simulink model "Euler_Quaternion"  (Simulink 7.9)
settings: Solver=ode45  StartTime=0.0  StopTime=10.0  RelTol=1e-3
undefined symbols (not defined in the file or in its folder): Newton, nfs, Raphson
libraries: aerolibanim x1, aerolibutil x1
settings Model: Creator=AHKh PC  LastModifiedBy=AHKh PC

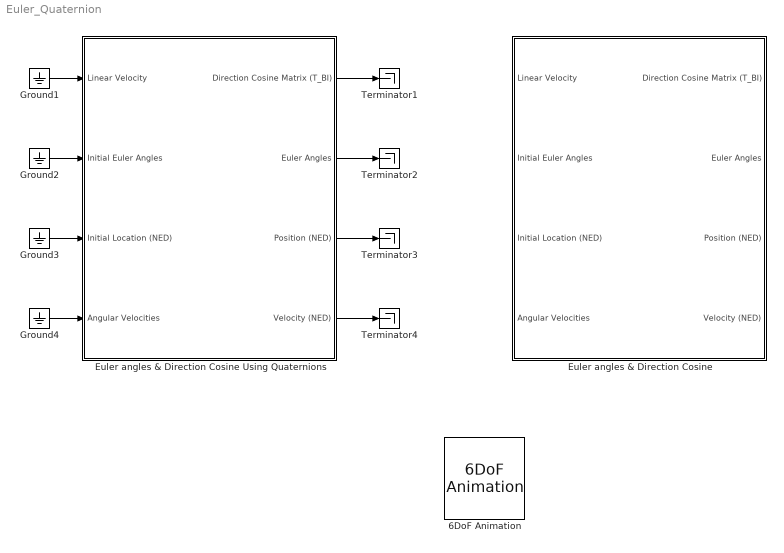
== system Euler_Quaternion ==
  6DoF Animation : aerolibanim/6DoF Animation  u1=[0 4000 -2000 2000 -5000 -3000]  u2=0.1  u3=1000.0  u4=[4000 0 -5000]  u5=Fly alongside  u6=[0 500 0]  u7=100  u8=on
  Euler angles & Direction Cosine : Subsystem
  Euler angles & Direction Cosine Using Quaternions : Subsystem
  Ground{1..4} (4 alike) : Ground
  Terminator{1..4} (4 alike) : Terminator
  wires:
  Euler angles & Direction Cosine Using Quaternions/1(Direction Cosine Matrix (T_BI)) -> Terminator1/1
  Euler angles & Direction Cosine Using Quaternions/2(Euler Angles) -> Terminator2/1
  Euler angles & Direction Cosine Using Quaternions/3(Position (NED)) -> Terminator3/1
  Euler angles & Direction Cosine Using Quaternions/4(Velocity (NED)) -> Terminator4/1
  Ground1/1 -> Euler angles & Direction Cosine Using Quaternions/1(Linear Velocity)
  Ground2/1 -> Euler angles & Direction Cosine Using Quaternions/2(Initial Euler Angles)
  Ground3/1 -> Euler angles & Direction Cosine Using Quaternions/3(Initial Location (NED))
  Ground4/1 -> Euler angles & Direction Cosine Using Quaternions/4(Angular Velocities)

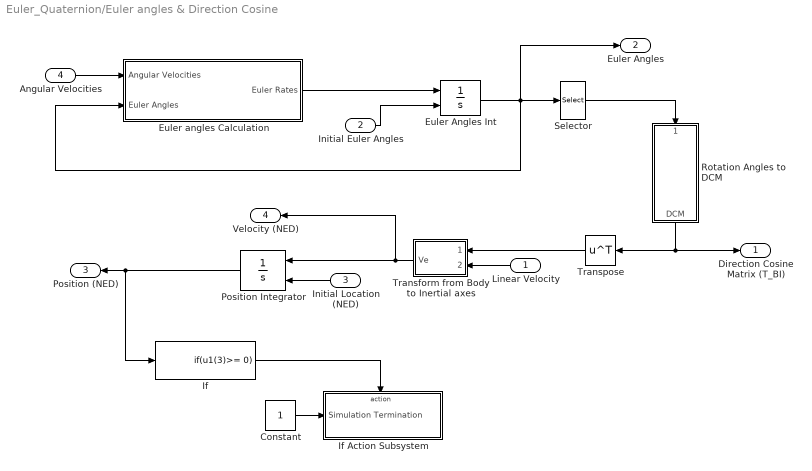
== system Euler_Quaternion/Euler angles & Direction Cosine ==
  Linear Velocity : Inport  PortDimensions=[3,1]
  Initial Euler Angles : Inport  Port=2
  Initial Location (NED) : Inport  Port=3  PortDimensions=[3,1]
  Angular Velocities : Inport  Port=4
  Constant : Constant
  Euler Angles Int : Integrator  InitialConditionSource=external  InitialCondition=nfs.attitude0
  Euler angles Calculation : Subsystem
  If : If  IfExpression=u1(3)>= 0  ShowElse=off
  If Action Subsystem : Subsystem  TreatAsAtomicUnit=on
  Position Integrator : Integrator  InitialConditionSource=external  InitialCondition=[0,0,nfs.attitude0]
  Rotation Angles to DCM : Subsystem
  Selector : Selector  InputPortWidth=3  IndexOptions=Index vector (dialog)  Indices=[3 2 1]  OutputSizes=1
  Transform from Body to Inertial axes : Subsystem
      mask Display: disp('T_IB')
  Transpose : Math  Operator=transpose  SaturateOnIntegerOverflow=on
  Direction Cosine Matrix (T_BI) : Outport  PortDimensions=[3,3]
  Euler Angles : Outport  Port=2
  Position (NED) : Outport  Port=3  PortDimensions=[3,1]
  Velocity (NED) : Outport  Port=4  PortDimensions=[3,1]
  wires:
  Initial Euler Angles/1 -> Euler Angles Int/2
  Rotation Angles to DCM/1(DCM) -> Transpose/1, Direction Cosine Matrix (T_BI)/1
  Angular Velocities/1 -> Euler angles Calculation/1(Angular Velocities)
  Selector/1 -> Rotation Angles to DCM/1("[R1,R2,R3]")
  Transpose/1 -> Transform from Body to Inertial axes/1(Transformation Matrix)
  Linear Velocity/1 -> Transform from Body to Inertial axes/2(Position Vector)
  Initial Location (NED)/1 -> Position Integrator/2
  Euler Angles Int/1 -> Euler Angles/1, Selector/1, Euler angles Calculation/2(Euler Angles)
  Transform from Body to Inertial axes/1(Ve) -> Velocity (NED)/1, Position Integrator/1
  Position Integrator/1 -> Position (NED)/1, If/1
  Euler angles Calculation/1(Euler Rates) -> Euler Angles Int/1
  If/1 -> If Action Subsystem/Action
  Constant/1 -> If Action Subsystem/1(Simulation Termination)

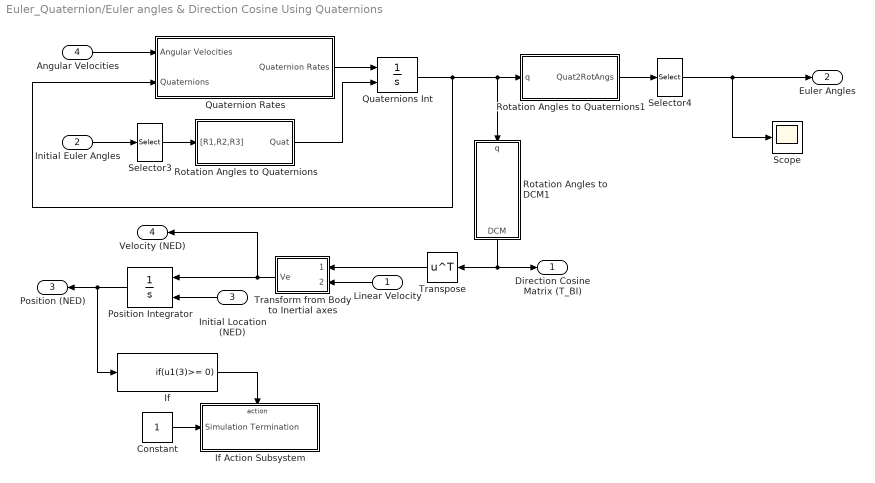
== system Euler_Quaternion/Euler angles & Direction Cosine Using Quaternions ==
  Linear Velocity : Inport  PortDimensions=[3,1]
  Initial Euler Angles : Inport  Port=2  PortDimensions=[3,1]
  Initial Location (NED) : Inport  Port=3  PortDimensions=[3,1]
  Angular Velocities : Inport  Port=4  PortDimensions=[3,1]
  Constant : Constant
  If : If  IfExpression=u1(3)>= 0  ShowElse=off
  If Action Subsystem : Subsystem  TreatAsAtomicUnit=on
  Position Integrator : Integrator  InitialConditionSource=external  InitialCondition=[0,0,nfs.attitude0]
  Quaternion Rates : Subsystem
  Quaternions Int : Integrator  InitialConditionSource=external  InitialCondition=nfs.attitude0  ContinuousStateAttributes='Quaternions'
  Rotation Angles to DCM1 : Subsystem
  Rotation Angles to Quaternions : Subsystem
  Rotation Angles to Quaternions1 : Subsystem
  Scope : Scope
      settings: SaveName=ScopeData23
  Selector3 : Selector  InputPortWidth=3  IndexOptions=Index vector (dialog)  Indices=[3 2 1]  OutputSizes=1
  Selector4 : Selector  InputPortWidth=3  IndexOptions=Index vector (dialog)  Indices=[3 2 1]  OutputSizes=1
  Transform from Body to Inertial axes : Subsystem
      mask Display: disp('T_IB')
  Transpose : Math  Operator=transpose  SaturateOnIntegerOverflow=on
  Direction Cosine Matrix (T_BI) : Outport  PortDimensions=[3,3]
  Euler Angles : Outport  Port=2  PortDimensions=[3,1]
  Position (NED) : Outport  Port=3  PortDimensions=[3,1]
  Velocity (NED) : Outport  Port=4  PortDimensions=[3,1]
  wires:
  Position Integrator/1 -> Position (NED)/1, If/1
  Transform from Body to Inertial axes/1(Ve) -> Position Integrator/1, Velocity (NED)/1
  Initial Location (NED)/1 -> Position Integrator/2
  Linear Velocity/1 -> Transform from Body to Inertial axes/2(Position Vector)
  Transpose/1 -> Transform from Body to Inertial axes/1(Transformation Matrix)
  Quaternion Rates/1(Quaternion Rates) -> Quaternions Int/1
  Angular Velocities/1 -> Quaternion Rates/1(Angular Velocities)
  Initial Euler Angles/1 -> Selector3/1
  Selector3/1 -> Rotation Angles to Quaternions/1("[R1,R2,R3]")
  Rotation Angles to Quaternions/1(Quat) -> Quaternions Int/2
  Quaternions Int/1 -> Quaternion Rates/2(Quaternions), Rotation Angles to Quaternions1/1(q), Rotation Angles to DCM1/1(q)
  Rotation Angles to Quaternions1/1(Quat2RotAngs) -> Selector4/1
  Selector4/1 -> Euler Angles/1, Scope/1
  Rotation Angles to DCM1/1(DCM) -> Direction Cosine Matrix (T_BI)/1, Transpose/1
  Constant/1 -> If Action Subsystem/1(Simulation Termination)
  If/1 -> If Action Subsystem/Action

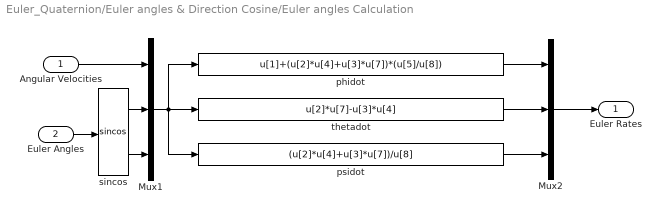
== system Euler_Quaternion/Euler angles & Direction Cosine/Euler angles Calculation ==
  Angular Velocities : Inport  PortDimensions=[3,1]
  Euler Angles : Inport  Port=2
  Mux1 : Mux  Inputs=[3 3 3]
  Mux2 : Mux  Inputs=3
  phidot : Fcn  Expr=u[1]+(u[2]*u[4]+u[3]*u[7])*(u[5]/u[8])
  psidot : Fcn  Expr=(u[2]*u[4]+u[3]*u[7])/u[8]
  sincos : Trigonometry  Operator=sincos
  thetadot : Fcn  Expr=u[2]*u[7]-u[3]*u[4]
  Euler Rates : Outport  PortDimensions=[3,1]  InitialOutput=0
  wires:
  sincos/2 -> Mux1/3
  sincos/1 -> Mux1/2
  Mux2/1 -> Euler Rates/1
  phidot/1 -> Mux2/1
  thetadot/1 -> Mux2/2
  psidot/1 -> Mux2/3
  Euler Angles/1 -> sincos/1
  Angular Velocities/1 -> Mux1/1
  Mux1/1 -> psidot/1, phidot/1, thetadot/1

== system Euler_Quaternion/Euler angles & Direction Cosine/If Action Subsystem ==
  Simulation Termination : Inport
  Action Port : ActionPort
  Stop Simulation : Stop
  wires:
  Simulation Termination/1 -> Stop Simulation/1

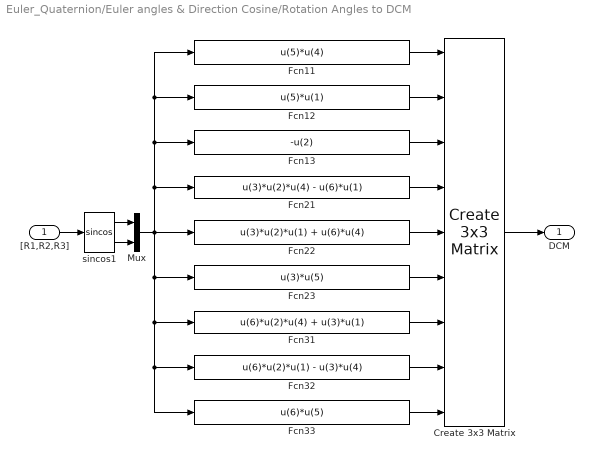
== system Euler_Quaternion/Euler angles & Direction Cosine/Rotation Angles to DCM ==
  "[R1,R2,R3]" : Inport  PortDimensions=3
  Create 3x3 Matrix : aerolibutil/Create 3x3 Matrix
  Fcn11 : Fcn  Expr=u(5)*u(4)
  Fcn12 : Fcn  Expr=u(5)*u(1)
  Fcn13 : Fcn  Expr=-u(2)
  Fcn21 : Fcn  Expr=u(3)*u(2)*u(4) - u(6)*u(1)
  Fcn22 : Fcn  Expr=u(3)*u(2)*u(1) + u(6)*u(4)
  Fcn23 : Fcn  Expr=u(3)*u(5)
  Fcn31 : Fcn  Expr=u(6)*u(2)*u(4) + u(3)*u(1)
  Fcn32 : Fcn  Expr=u(6)*u(2)*u(1) - u(3)*u(4)
  Fcn33 : Fcn  Expr=u(6)*u(5)
  Mux : Mux  Inputs=2
  sincos1 : Trigonometry  Operator=sincos
  DCM : Outport  PortDimensions=[3,3]
  wires:
  "[R1,R2,R3]"/1 -> sincos1/1
  Create 3x3 Matrix/1 -> DCM/1
  sincos1/1 -> Mux/1
  sincos1/2 -> Mux/2
  Mux/1 -> Fcn32/1, Fcn33/1, Fcn31/1, Fcn23/1, Fcn22/1, Fcn11/1, Fcn12/1, Fcn13/1, Fcn21/1
  Fcn11/1 -> Create 3x3 Matrix/1
  Fcn12/1 -> Create 3x3 Matrix/2
  Fcn13/1 -> Create 3x3 Matrix/3
  Fcn21/1 -> Create 3x3 Matrix/4
  Fcn31/1 -> Create 3x3 Matrix/7
  Fcn22/1 -> Create 3x3 Matrix/5
  Fcn23/1 -> Create 3x3 Matrix/6
  Fcn32/1 -> Create 3x3 Matrix/8
  Fcn33/1 -> Create 3x3 Matrix/9

== system Euler_Quaternion/Euler angles & Direction Cosine/Transform from Body to Inertial axes ==
  Transformation Matrix : Inport
  Position Vector : Inport  Port=2
  Product : Product  Multiplication=Matrix(*)  SaturateOnIntegerOverflow=on  InputSameDT=on  OutDataTypeStr=Inherit: Same as first input
  Reshape1 : Reshape  OutputDimensionality=Column vector (2-D)
  Reshape2 : Reshape
  Ve : Outport
  wires:
  Reshape2/1 -> Ve/1
  Reshape1/1 -> Product/2
  Position Vector/1 -> Reshape1/1
  Transformation Matrix/1 -> Product/1
  Product/1 -> Reshape2/1

== system Euler_Quaternion/Euler angles & Direction Cosine Using Quaternions/If Action Subsystem ==
  Simulation Termination : Inport
  Action Port : ActionPort  ActionType=then
  Stop Simulation : Stop
  wires:
  Simulation Termination/1 -> Stop Simulation/1

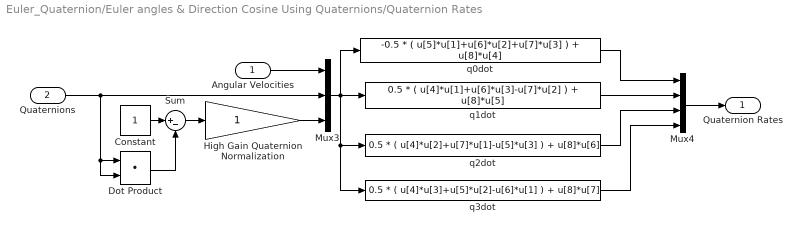
== system Euler_Quaternion/Euler angles & Direction Cosine Using Quaternions/Quaternion Rates ==
  Angular Velocities : Inport  PortDimensions=[3,1]
  Quaternions : Inport  Port=2  PortDimensions=4
  Constant : Constant
  Dot Product : DotProduct  OutDataTypeStr=Inherit: Inherit via internal rule
  High Gain Quaternion Normalization : Gain  SaturateOnIntegerOverflow=on  OutDataTypeStr=Inherit: Same as input  ParamDataTypeStr=Inherit: Same as input
  Mux3 : Mux  Inputs=[3 4 1]
  Mux4 : Mux
  Sum : Sum  Inputs=|+-  SaturateOnIntegerOverflow=on  InputSameDT=on  OutDataTypeStr=Inherit: Same as first input
  q0dot : Fcn  Expr=-0.5 * ( u[5]*u[1]+u[6]*u[2]+u[7]*u[3] ) + u[8]*u[4]
  q1dot : Fcn  Expr=0.5 * ( u[4]*u[1]+u[6]*u[3]-u[7]*u[2] ) + u[8]*u[5]
  q2dot : Fcn  Expr=0.5 * ( u[4]*u[2]+u[7]*u[1]-u[5]*u[3] ) + u[8]*u[6]
  q3dot : Fcn  Expr=0.5 * ( u[4]*u[3]+u[5]*u[2]-u[6]*u[1] ) + u[8]*u[7]
  Quaternion Rates : Outport  PortDimensions=4  InitialOutput=0
  wires:
  Angular Velocities/1 -> Mux3/1
  Dot Product/1 -> Sum/2
  High Gain Quaternion Normalization/1 -> Mux3/3
  Sum/1 -> High Gain Quaternion Normalization/1
  Constant/1 -> Sum/1
  Mux4/1 -> Quaternion Rates/1
  q0dot/1 -> Mux4/1
  q1dot/1 -> Mux4/2
  q2dot/1 -> Mux4/3
  Mux3/1 -> q2dot/1, q3dot/1, q0dot/1, q1dot/1
  q3dot/1 -> Mux4/4
  Quaternions/1 -> Dot Product/1, Dot Product/2, Mux3/2

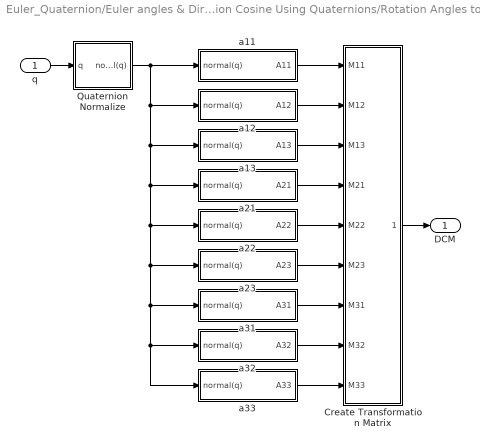
== system Euler_Quaternion/Euler angles & Direction Cosine Using Quaternions/Rotation Angles to DCM1 ==
  q : Inport  PortDimensions=4
  Create Transformation Matrix : Subsystem
  Quaternion Normalize : Subsystem
  a11 : Subsystem
  a12 : Subsystem
  a13 : Subsystem
  a21 : Subsystem
  a22 : Subsystem
  a23 : Subsystem
  a31 : Subsystem
  a32 : Subsystem
  a33 : Subsystem
  DCM : Outport  PortDimensions=[3,3]
  wires:
  q/1 -> Quaternion Normalize/1(q)
  a11/1(A11) -> Create Transformation Matrix/1(M11)
  a12/1(A12) -> Create Transformation Matrix/2(M12)
  a13/1(A13) -> Create Transformation Matrix/3(M13)
  a21/1(A21) -> Create Transformation Matrix/4(M21)
  a22/1(A22) -> Create Transformation Matrix/5(M22)
  a23/1(A23) -> Create Transformation Matrix/6(M23)
  a31/1(A31) -> Create Transformation Matrix/7(M31)
  a32/1(A32) -> Create Transformation Matrix/8(M32)
  a33/1(A33) -> Create Transformation Matrix/9(M33)
  Quaternion Normalize/1(normal(q)) -> a33/1(normal(q)), a32/1(normal(q)), a31/1(normal(q)), a23/1(normal(q)), a22/1(normal(q)), a21/1(normal(q)), a13/1(normal(q)), a12/1(normal(q)), a11/1(normal(q))
  Create Transformation Matrix/1(Matrix) -> DCM/1

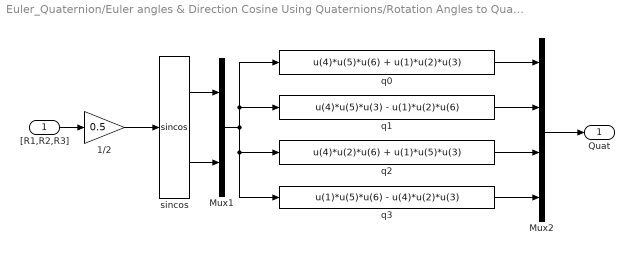
== system Euler_Quaternion/Euler angles & Direction Cosine Using Quaternions/Rotation Angles to Quaternions ==
  "[R1,R2,R3]" : Inport  PortDimensions=3
  1/2 : Gain  Gain=0.5  SaturateOnIntegerOverflow=on  OutDataTypeStr=Inherit: Same as input  ParamDataTypeStr=Inherit: Same as input
  Mux1 : Mux  Inputs=2
  Mux2 : Mux
  q0 : Fcn  Expr=u(4)*u(5)*u(6) + u(1)*u(2)*u(3)
  q1 : Fcn  Expr=u(4)*u(5)*u(3) - u(1)*u(2)*u(6)
  q2 : Fcn  Expr=u(4)*u(2)*u(6) + u(1)*u(5)*u(3)
  q3 : Fcn  Expr=u(1)*u(5)*u(6) - u(4)*u(2)*u(3)
  sincos : Trigonometry  Operator=sincos
  Quat : Outport  PortDimensions=4
  wires:
  q0/1 -> Mux2/1
  Mux2/1 -> Quat/1
  q3/1 -> Mux2/4
  q2/1 -> Mux2/3
  q1/1 -> Mux2/2
  Mux1/1 -> q3/1, q2/1, q1/1, q0/1
  sincos/2 -> Mux1/2
  sincos/1 -> Mux1/1
  1/2/1 -> sincos/1
  "[R1,R2,R3]"/1 -> 1/2/1

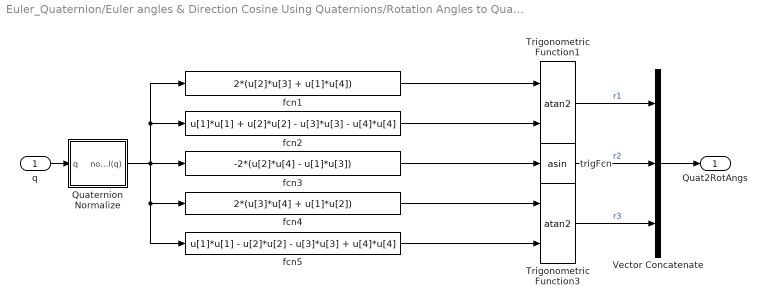
== system Euler_Quaternion/Euler angles & Direction Cosine Using Quaternions/Rotation Angles to Quaternions1 ==
  q : Inport  PortDimensions=4
  Quaternion Normalize : Subsystem
  Trigonometric Function1 : Trigonometry  Operator=atan2
  Trigonometric Function3 : Trigonometry  Operator=atan2
  Vector Concatenate : Concatenate  NumInputs=3
  fcn1 : Fcn  Expr=2*(u[2]*u[3] + u[1]*u[4])
  fcn2 : Fcn  Expr=u[1]*u[1] + u[2]*u[2] - u[3]*u[3] - u[4]*u[4]
  fcn3 : Fcn  Expr=-2*(u[2]*u[4] - u[1]*u[3])
  fcn4 : Fcn  Expr=2*(u[3]*u[4] + u[1]*u[2])
  fcn5 : Fcn  Expr=u[1]*u[1] - u[2]*u[2] - u[3]*u[3] + u[4]*u[4]
  trigFcn : Trigonometry  Operator=asin
  Quat2RotAngs : Outport  PortDimensions=[3,1]
  wires:
  fcn5/1 -> Trigonometric Function3/2
  fcn4/1 -> Trigonometric Function3/1
  fcn2/1 -> Trigonometric Function1/2
  fcn1/1 -> Trigonometric Function1/1
  fcn3/1 -> trigFcn/1
  Trigonometric Function1/1 -> Vector Concatenate/1  "r1"
  trigFcn/1 -> Vector Concatenate/2  "r2"
  Trigonometric Function3/1 -> Vector Concatenate/3  "r3"
  Quaternion Normalize/1(normal(q)) -> fcn1/1, fcn2/1, fcn5/1, fcn4/1, fcn3/1
  q/1 -> Quaternion Normalize/1(q)
  Vector Concatenate/1 -> Quat2RotAngs/1

== system Euler_Quaternion/Euler angles & Direction Cosine Using Quaternions/Transform from Body to Inertial axes ==
  Transformation Matrix : Inport
  Position Vector : Inport  Port=2
  Product : Product  Multiplication=Matrix(*)  SaturateOnIntegerOverflow=on  InputSameDT=on  OutDataTypeStr=Inherit: Same as first input
  Reshape1 : Reshape  OutputDimensionality=Column vector (2-D)
  Reshape2 : Reshape
  Ve : Outport
  wires:
  Product/1 -> Reshape2/1
  Transformation Matrix/1 -> Product/1
  Position Vector/1 -> Reshape1/1
  Reshape1/1 -> Product/2
  Reshape2/1 -> Ve/1

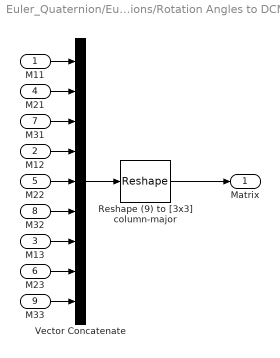
== system Euler_Quaternion/Euler angles & Direction Cosine Using Quaternions/Rotation Angles to DCM1/Create Transformation Matrix ==
  M11 : Inport  PortDimensions=1
  M12 : Inport  Port=2  PortDimensions=1
  M13 : Inport  Port=3  PortDimensions=1
  M21 : Inport  Port=4  PortDimensions=1
  M22 : Inport  Port=5  PortDimensions=1
  M23 : Inport  Port=6  PortDimensions=1
  M31 : Inport  Port=7  PortDimensions=1
  M32 : Inport  Port=8  PortDimensions=1
  M33 : Inport  Port=9  PortDimensions=1
  Reshape (9) to [3x3] column-major : Reshape  OutputDimensionality=Customize  OutputDimensions=[3,3]
  Vector Concatenate : Concatenate  NumInputs=9
  Matrix : Outport  PortDimensions=[3 3]
  wires:
  M33/1 -> Vector Concatenate/9
  M23/1 -> Vector Concatenate/8
  M13/1 -> Vector Concatenate/7
  M32/1 -> Vector Concatenate/6
  Reshape (9) to [3x3] column-major/1 -> Matrix/1
  M22/1 -> Vector Concatenate/5
  M12/1 -> Vector Concatenate/4
  M31/1 -> Vector Concatenate/3
  M21/1 -> Vector Concatenate/2
  M11/1 -> Vector Concatenate/1
  Vector Concatenate/1 -> Reshape (9) to [3x3] column-major/1

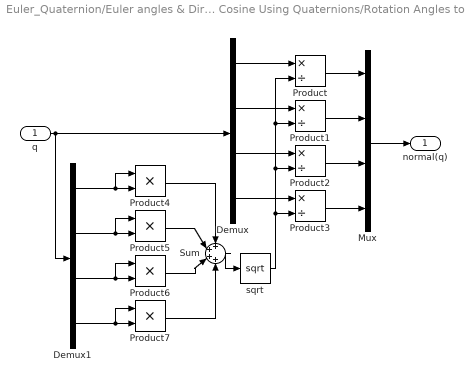
== system Euler_Quaternion/Euler angles & Direction Cosine Using Quaternions/Rotation Angles to DCM1/Quaternion Normalize ==
  q : Inport
  Demux : Demux
  Demux1 : Demux
  Mux : Mux
  Product{,1..3} (4 alike) : Product  Inputs=*/
  Product{4..7} (4 alike) : Product
  Sum : Sum  Inputs=4
  sqrt : Sqrt  AlgorithmType=Newton-Raphson  SaturateOnIntegerOverflow=on
  normal(q) : Outport
  wires:
  Product3/1 -> Mux/4
  Product2/1 -> Mux/3
  Product1/1 -> Mux/2
  Product/1 -> Mux/1
  sqrt/1 -> Product3/2, Product2/2, Product/2, Product1/2
  q/1 -> Demux/1, Demux1/1
  Mux/1 -> normal(q)/1
  Demux/1 -> Product/1
  Demux/2 -> Product1/1
  Demux/3 -> Product2/1
  Demux/4 -> Product3/1
  Sum/1 -> sqrt/1
  Product4/1 -> Sum/1
  Product5/1 -> Sum/2
  Product6/1 -> Sum/3
  Product7/1 -> Sum/4
  Demux1/1 -> Product4/2, Product4/1
  Demux1/2 -> Product5/2, Product5/1
  Demux1/3 -> Product6/2, Product6/1
  Demux1/4 -> Product7/2, Product7/1

== system Euler_Quaternion/Euler angles & Direction Cosine Using Quaternions/Rotation Angles to DCM1/a11 ==
  normal(q) : Inport
  Demux : Demux
  Product{,1..3} (4 alike) : Product  RndMeth=Zero
  Sum : Sum  Inputs=++--
  A11 : Outport
  wires:
  Sum/1 -> A11/1
  Demux/4 -> Product/2, Product/1
  Demux/3 -> Product1/2, Product1/1
  Demux/2 -> Product2/2, Product2/1
  Demux/1 -> Product3/2, Product3/1
  Product3/1 -> Sum/1
  Product2/1 -> Sum/2
  Product1/1 -> Sum/3
  Product/1 -> Sum/4
  normal(q)/1 -> Demux/1

== system Euler_Quaternion/Euler angles & Direction Cosine Using Quaternions/Rotation Angles to DCM1/a12 ==
  normal(q) : Inport
  Demux : Demux
  Gain : Gain  Gain=2
  Product2 : Product  RndMeth=Zero
  Product3 : Product  RndMeth=Zero
  Sum : Sum  Inputs=|++
  A12 : Outport
  wires:
  Product2/1 -> Sum/2
  Product3/1 -> Sum/1
  Sum/1 -> Gain/1
  Demux/1 -> Product3/2
  Demux/2 -> Product2/1
  Demux/4 -> Product3/1
  Demux/3 -> Product2/2
  normal(q)/1 -> Demux/1
  Gain/1 -> A12/1

== system Euler_Quaternion/Euler angles & Direction Cosine Using Quaternions/Rotation Angles to DCM1/a13 ==
  normal(q) : Inport
  Demux : Demux
  Gain : Gain  Gain=2
  Product1 : Product  RndMeth=Zero
  Product2 : Product  RndMeth=Zero
  Sum : Sum  Inputs=|-+
  A13 : Outport
  wires:
  Demux/1 -> Product1/1
  Product1/1 -> Sum/1
  Product2/1 -> Sum/2
  Demux/4 -> Product2/2
  Demux/2 -> Product2/1
  Demux/3 -> Product1/2
  normal(q)/1 -> Demux/1
  Gain/1 -> A13/1
  Sum/1 -> Gain/1

== system Euler_Quaternion/Euler angles & Direction Cosine Using Quaternions/Rotation Angles to DCM1/a21 ==
  normal(q) : Inport
  Demux : Demux
  Gain : Gain  Gain=2
  Product2 : Product  RndMeth=Zero
  Product3 : Product  RndMeth=Zero
  Sum : Sum  Inputs=|-+
  A21 : Outport
  wires:
  Gain/1 -> A21/1
  normal(q)/1 -> Demux/1
  Demux/3 -> Product2/2
  Demux/4 -> Product3/1
  Demux/2 -> Product2/1
  Demux/1 -> Product3/2
  Sum/1 -> Gain/1
  Product3/1 -> Sum/1
  Product2/1 -> Sum/2

== system Euler_Quaternion/Euler angles & Direction Cosine Using Quaternions/Rotation Angles to DCM1/a22 ==
  normal(q) : Inport
  Demux : Demux
  Product{,1..3} (4 alike) : Product  RndMeth=Zero
  Sum : Sum  Inputs=+-+-
  A22 : Outport
  wires:
  normal(q)/1 -> Demux/1
  Product/1 -> Sum/4
  Product1/1 -> Sum/3
  Product2/1 -> Sum/2
  Product3/1 -> Sum/1
  Demux/1 -> Product3/1, Product3/2
  Demux/2 -> Product2/1, Product2/2
  Demux/3 -> Product1/1, Product1/2
  Demux/4 -> Product/1, Product/2
  Sum/1 -> A22/1

== system Euler_Quaternion/Euler angles & Direction Cosine Using Quaternions/Rotation Angles to DCM1/a23 ==
  normal(q) : Inport
  Demux : Demux
  Gain : Gain  Gain=2
  Product1 : Product  RndMeth=Zero
  Product2 : Product  RndMeth=Zero
  Sum : Sum  Inputs=|++
  A23 : Outport
  wires:
  Demux/4 -> Product2/2
  Product2/1 -> Sum/2
  Product1/1 -> Sum/1
  Sum/1 -> Gain/1
  Demux/1 -> Product1/1
  Demux/2 -> Product1/2
  Demux/3 -> Product2/1
  Gain/1 -> A23/1
  normal(q)/1 -> Demux/1

== system Euler_Quaternion/Euler angles & Direction Cosine Using Quaternions/Rotation Angles to DCM1/a31 ==
  normal(q) : Inport
  Demux : Demux
  Gain : Gain  Gain=2
  Product1 : Product  RndMeth=Zero
  Product2 : Product  RndMeth=Zero
  Sum : Sum  Inputs=|++
  A31 : Outport
  wires:
  Sum/1 -> Gain/1
  Gain/1 -> A31/1
  normal(q)/1 -> Demux/1
  Demux/3 -> Product1/2
  Demux/2 -> Product2/1
  Demux/4 -> Product2/2
  Product2/1 -> Sum/2
  Product1/1 -> Sum/1
  Demux/1 -> Product1/1

== system Euler_Quaternion/Euler angles & Direction Cosine Using Quaternions/Rotation Angles to DCM1/a32 ==
  normal(q) : Inport
  Demux : Demux
  Gain : Gain  Gain=2
  Product1 : Product  RndMeth=Zero
  Product2 : Product  RndMeth=Zero
  Sum : Sum  Inputs=|-+
  A32 : Outport
  wires:
  normal(q)/1 -> Demux/1
  Gain/1 -> A32/1
  Demux/3 -> Product2/1
  Demux/2 -> Product1/2
  Demux/1 -> Product1/1
  Sum/1 -> Gain/1
  Product1/1 -> Sum/1
  Product2/1 -> Sum/2
  Demux/4 -> Product2/2

== system Euler_Quaternion/Euler angles & Direction Cosine Using Quaternions/Rotation Angles to DCM1/a33 ==
  normal(q) : Inport
  Demux : Demux
  Product{,1..3} (4 alike) : Product  RndMeth=Zero
  Sum : Sum  Inputs=+--+
  A33 : Outport
  wires:
  normal(q)/1 -> Demux/1
  Product/1 -> Sum/4
  Product1/1 -> Sum/3
  Product2/1 -> Sum/2
  Product3/1 -> Sum/1
  Demux/1 -> Product3/1, Product3/2
  Demux/2 -> Product2/1, Product2/2
  Demux/3 -> Product1/1, Product1/2
  Demux/4 -> Product/1, Product/2
  Sum/1 -> A33/1

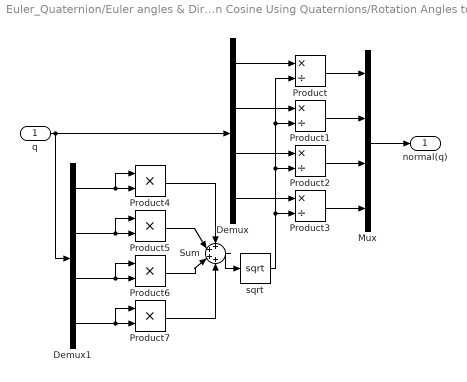
== system Euler_Quaternion/Euler angles & Direction Cosine Using Quaternions/Rotation Angles to Quaternions1/Quaternion Normalize ==
  q : Inport
  Demux : Demux
  Demux1 : Demux
  Mux : Mux
  Product{,1..3} (4 alike) : Product  Inputs=*/
  Product{4..7} (4 alike) : Product
  Sum : Sum  Inputs=4
  sqrt : Sqrt  AlgorithmType=Newton-Raphson  SaturateOnIntegerOverflow=on
  normal(q) : Outport
  wires:
  Product3/1 -> Mux/4
  Product2/1 -> Mux/3
  Product1/1 -> Mux/2
  Product/1 -> Mux/1
  sqrt/1 -> Product3/2, Product2/2, Product/2, Product1/2
  q/1 -> Demux/1, Demux1/1
  Mux/1 -> normal(q)/1
  Demux/1 -> Product/1
  Demux/2 -> Product1/1
  Demux/3 -> Product2/1
  Demux/4 -> Product3/1
  Sum/1 -> sqrt/1
  Product4/1 -> Sum/1
  Product5/1 -> Sum/2
  Product6/1 -> Sum/3
  Product7/1 -> Sum/4
  Demux1/1 -> Product4/2, Product4/1
  Demux1/2 -> Product5/2, Product5/1
  Demux1/3 -> Product6/2, Product6/1
  Demux1/4 -> Product7/2, Product7/1
